simulink library "combinedController_cl"  (R2018b)
settings: Solver=VariableStepAuto  StartTime=0.0  StopTime=10.0  RelTol=1e-3
libraries: pathFollowingController_cl x1, courseFollow_cl x1
settings Model: Creator=jldanie5  LastModifiedBy=jldanie5

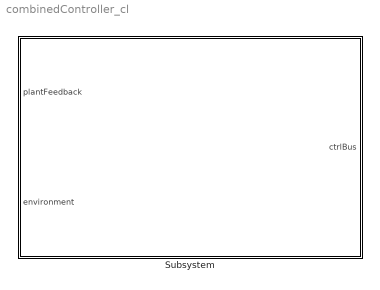
== system combinedController_cl ==
  Subsystem : Subsystem  mask{a_user=0, b_user=0, phiG_user=0, path_user=0, S_user=0}
      mask prompts: a_user "Path Param A"; b_user "Path Param B"; phiG_user "PhiG"; path_user "Path"; S_user "S"

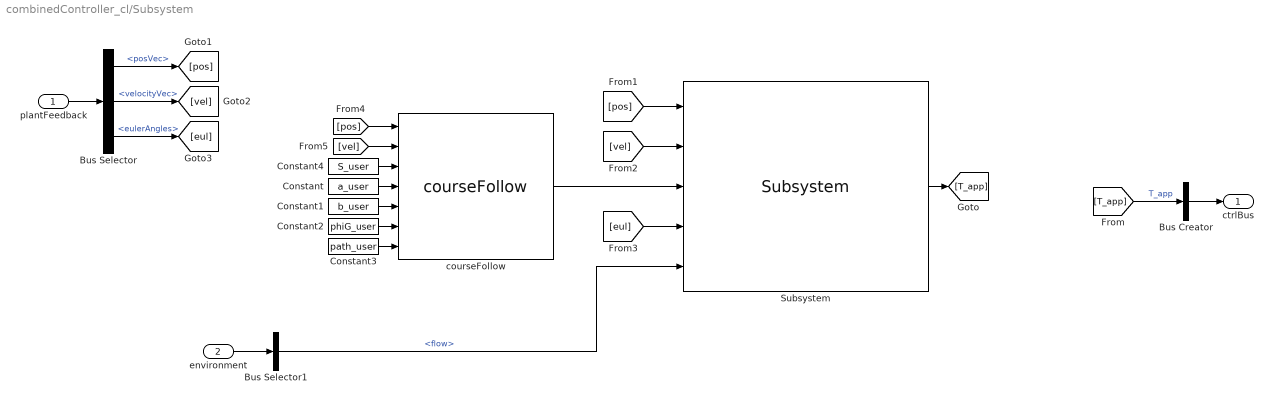
== system combinedController_cl/Subsystem ==
  plantFeedback : Inport  OutDataTypeStr=Bus: plantBus
  environment : Inport  Port=2  OutDataTypeStr=Bus: envBus
  Bus Creator : BusCreator  Inputs=1  OutDataTypeStr=Bus: ctrlBus
  Bus Selector : BusSelector  OutputSignals=posVec,velocityVec,eulerAngles
  Bus Selector1 : BusSelector  OutputSignals=flow
  Constant : Constant  Value=a_user
  Constant1 : Constant  Value=b_user
  Constant2 : Constant  Value=phiG_user
  Constant3 : Constant  Value=path_user
  Constant4 : Constant  Value=S_user
  Subsystem : pathFollowingController_cl/Subsystem  AoA_des=0  controlMat=0  ctrlSigMax=0
  courseFollow : courseFollow_cl/courseFollow  SystemSampleTime=-1
  ctrlBus : Outport
  wires:
  Subsystem/1 -> [T_app]
  courseFollow/1 -> Subsystem/3
  Bus Creator/1 -> ctrlBus/1
  Bus Selector1/1 -> Subsystem/5  "<flow>"
  environment/1 -> Bus Selector1/1
  plantFeedback/1 -> Bus Selector/1
  Bus Selector/2 -> [vel]  "<velocityVec>"
  Bus Selector/1 -> [pos]  "<posVec>"
  Bus Selector/3 -> [eul]  "<eulerAngles>"
  [pos] -> Subsystem/1
  [vel] -> Subsystem/2
  [eul] -> Subsystem/4
  [T_app] -> Bus Creator/1  "T_app"
  [pos] -> courseFollow/1
  [vel] -> courseFollow/2
  Constant/1 -> courseFollow/4
  Constant1/1 -> courseFollow/5
  Constant3/1 -> courseFollow/7
  Constant2/1 -> courseFollow/6
  Constant4/1 -> courseFollow/3
